simulink model "model2"  (R2023b)
settings: Solver=VariableStepAuto  StartTime=1  StopTime=2  RelTol=1e-3
undefined symbols (not defined in the file): DiscIntNeverNeededParam
settings Model: Creator=Антон  LastModifiedBy=OskolockKoli

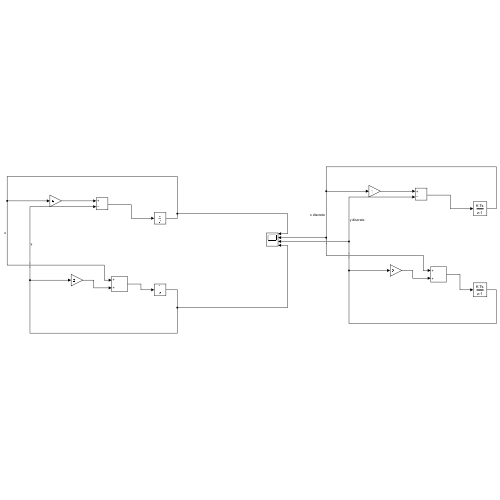
[thumbnail: Simulink's stored preview of the top-level diagram]
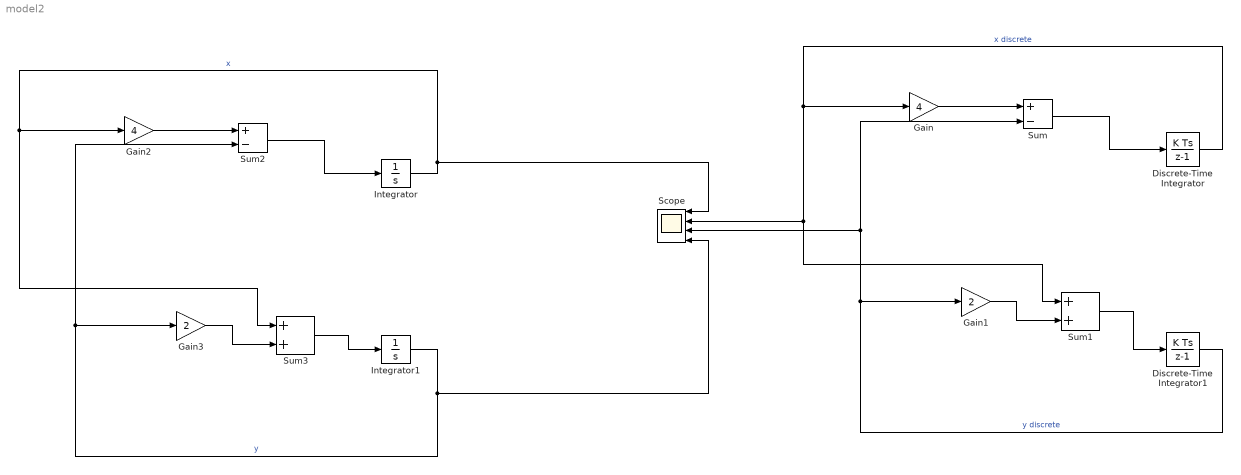
== system model2 ==
  Discrete-Time Integrator : DiscreteIntegrator  InitialCondition=-2  SampleTime=0.05  ICPrevOutput=DiscIntNeverNeededParam  ICPrevScaledInput=DiscIntNeverNeededParam
  Discrete-Time Integrator1 : DiscreteIntegrator  SampleTime=0.05  ICPrevOutput=DiscIntNeverNeededParam  ICPrevScaledInput=DiscIntNeverNeededParam
  Gain : Gain  Gain=4
  Gain1 : Gain  Gain=2
  Gain2 : Gain  Gain=4
  Gain3 : Gain  Gain=2
  Integrator : Integrator  InitialCondition=-2
  Integrator1 : Integrator
  Scope : Scope  NumInputPorts=4
  Sum : Sum  Inputs=+-
  Sum1 : Sum
  Sum2 : Sum  Inputs=+-
  Sum3 : Sum
  wires:
  Discrete-Time Integrator/1 -> Sum1/1, Scope/2, Gain/1  "x discrete"
  Discrete-Time Integrator1/1 -> Sum/2, Scope/3, Gain1/1  "y discrete"
  Gain/1 -> Sum/1
  Sum/1 -> Discrete-Time Integrator/1
  Gain1/1 -> Sum1/2
  Sum1/1 -> Discrete-Time Integrator1/1
  Gain3/1 -> Sum3/2
  Gain2/1 -> Sum2/1
  Sum3/1 -> Integrator1/1
  Integrator1/1 -> Scope/4, Sum2/2, Gain3/1  "y"
  Integrator/1 -> Scope/1, Sum3/1, Gain2/1  "x"
  Sum2/1 -> Integrator/1
